simulink model "ofdm_agc_mimo"  (Simulink 7.7)
settings: Solver=VariableStepDiscrete  SolverMode=SingleTasking  StartTime=0.0  StopTime=400  RelTol=1e-3
InitFcn:
  | ofdm_agc_init
StartFcn:
  | ofdm_agc_init
values from neighbouring files (symbols this model uses):
  ltbl = ltbl(2:2049)    [ofdm_agc_init.m]
undefined symbols (not defined in the file or in its folder): gcbh, xlBlockLoadCallback, xlGetNormalizedPeriod
libraries: xbsIndex_r4 x570
(part 5 of 6)

== system ofdm_agc_mimo/Dual_channel_VIQ/AVG_I_Q3 ==
  note: Calculates the average of the I and Q channels, before taking the CPLX mag
  RESET : Inport
  CPLX_in : Inport  Port=2
  IQAvg_Len : Inport  Port=3
  ASR_I : xbsIndex_r4/Addressable Shift Register  infer_latency=on  depth=2  initVector=[0]  en=off  dbl_ovrd=off  use_behavioral_HDL=off  Optimization=Resource  use_rpm=off  block_type=addrsr
      settings: infoedit="Delay of  configurable length.  Any element  in the delay     line   can    be   addressed   and   driven    onto   the   output     port.<P><P>Hardware  notes: Implemented  using SRL16s.     If Virtex-4, Virtex-II or Spartan-3 devices are used, multiple SRLC16s are cascaded together."  xl_area=[51 0 0 102 0 0 0]  block_version=VER_STRING_GOES_HERE
  Accumulator : xbsIndex_r4/Accumulator  operation=Add  n_bits=24  overflow=Wrap  scale=1  rst=on  hasbypass=off  en=off  dbl_ovrd=off  use_behavioral_HDL=on  implementation=Fabric  block_type=accum
      settings: infoedit="Adder or subtractor-based accumulator.   Output type and binary point position match the input.<P><P>Hardware notes: When \"Reinitialize with input 'b' on reset\" is selected, the accumulator is forced to run at the system rate even if the input 'b' is running at a slower rate."  xl_area=[12 24 0 24 0 0 0]  block_version=VER_STRING_GOES_HERE
  AddSub : xbsIndex_r4/AddSub  mode=Addition  use_carryin=off  use_carryout=off  en=off  latency=0  precision=Full  arith_type=Unsigned  n_bits=8  bin_pt=2  quantization=Truncate  overflow=Wrap  dbl_ovrd=off  use_behavioral_HDL=on  hw_selection=Fabric  pipelined=off  use_rpm=on  block_type=addsub
      settings: xl_area=[10 0 0 18 0 0 0]  block_version=VER_STRING_GOES_HERE
  Convert : xbsIndex_r4/Convert  gui_display_data_type=Fixed-point  arith_type="Signed  (2's comp)"  n_bits=24  bin_pt=16  float_type=Single  exp_bits=8  fraction_bits=24  quantization=Truncate  overflow=Wrap  en=off  latency=0  dbl_ovrd=off  pipeline=off  block_type=convert
      settings: xl_area=[0 0 0 0 0 0 0]  block_version=VER_STRING_GOES_HERE
  Convert1 : xbsIndex_r4/Convert  gui_display_data_type=Fixed-point  arith_type=Unsigned  n_bits=6  bin_pt=0  float_type=Single  exp_bits=8  fraction_bits=24  quantization=Truncate  overflow=Wrap  en=off  latency=0  dbl_ovrd=off  pipeline=off  block_type=convert
      settings: xl_area=[0 0 0 0 0 0 0]  block_version=VER_STRING_GOES_HERE
  Down Sample3 : xbsIndex_r4/Down Sample  sample_ratio=4  sample_phase="Last Value of Frame  (most efficient)"  en=off  latency=1  dbl_ovrd=off  block_type=dsamp
      settings: xl_area=[3 6 0 0 0 0 0]  block_version=VER_STRING_GOES_HERE
  Mult : xbsIndex_r4/Mult  precision=User Defined  arith_type="Signed  (2's comp)"  n_bits=16  bin_pt=13  quantization=Truncate  overflow=Wrap  en=off  latency=3  dbl_ovrd=off  use_behavioral_HDL=off  opt=Speed  use_embedded=on  optimum_pipeline=off  pipeline=on  use_rpm=on  placement_style=Rectangular shape  block_type=mult
      settings: infoedit=Hardware notes: To use the internal pipeline stage of the dedicated multiplier you must select 'Pipeline for maximum performance'.  xl_area=[21 41 0 35 0 2 0]  block_version=VER_STRING_GOES_HERE
  Negate_I : xbsIndex_r4/Negate  precision=Full  arith_type=Unsigned  n_bits=8  bin_pt=2  quantization=Truncate  overflow=Wrap  en=off  latency=0  dbl_ovrd=off  block_type=negate
      settings: xl_area=[9 0 0 18 0 0 0]  block_version=VER_STRING_GOES_HERE
  Register15 : xbsIndex_r4/Register  init=0  rst=on  en=off  dbl_ovrd=off  block_type=register
      settings: xl_area=[9 17 0 0 0 0 0]  block_version=VER_STRING_GOES_HERE
  one_over_delay : xbsIndex_r4/ROM  depth=64  initVector=[1./(1:64)]  distributed_mem=Block RAM  rst=off  init_reg=0  en=off  latency=1  gui_display_data_type=Fixed-point  arith_type=Unsigned  n_bits=8  bin_pt=8  preci_type=Single  exp_width=8  frac_width=24  dbl_ovrd=off  optimize=Area  use_rpm=off  block_type=sprom
      settings: xl_area=[8 8 0 16 0 0 0]  block_version=VER_STRING_GOES_HERE
  AVG_CPLX_out : Outport
  wires:
  RESET/1 -> Accumulator/2, Register15/2
  Register15/1 -> AddSub/1, ASR_I/1
  Convert/1 -> Accumulator/1
  Negate_I/1 -> AddSub/2
  AddSub/1 -> Convert/1
  Mult/1 -> AVG_CPLX_out/1
  IQAvg_Len/1 -> Down Sample3/1
  one_over_delay/1 -> Mult/2
  Accumulator/1 -> Mult/1
  ASR_I/1 -> Negate_I/1
  CPLX_in/1 -> Register15/1
  Down Sample3/1 -> ASR_I/2, Convert1/1
  Convert1/1 -> one_over_delay/1

== system ofdm_agc_mimo/Dual_channel_VIQ/Timeshared_squarer ==
  note: Squares four parallel streams of data
  I_A : Inport
  Q_A : Inport  Port=2
  I_B : Inport  Port=3
  Q_B : Inport  Port=4
  Convert1 : xbsIndex_r4/Convert  gui_display_data_type=Fixed-point  arith_type=Unsigned  n_bits=16  bin_pt=13  float_type=Single  exp_bits=8  fraction_bits=24  quantization="Round  (unbiased: +/- Inf)"  overflow=Wrap  en=off  latency=0  dbl_ovrd=off  pipeline=off  block_type=convert
      settings: xl_area=[13 0 0 20 0 0 0]  block_version=VER_STRING_GOES_HERE
  Delay : xbsIndex_r4/Delay  rst=off  infoeditControl=Selection of Reset will increase slice count due to use of real FFs and instead of SRLs  en=off  latency=1  dbl_ovrd=off  reg_retiming=off  block_type=delay
      settings: infoedit=Hardware notes: A delay line is a chain, each link of which is an SRL16 followed by a flip-flop. If register retiming is enabled, the delay line is a chain of flip-flops.  xl_area=[8 16 0 0 0 0 0]  block_version=VER_STRING_GOES_HERE
  Down Sample{,1..3} (4 alike) : xbsIndex_r4/Down Sample  sample_ratio=4  sample_phase="Last Value of Frame  (most efficient)"  en=off  latency=1  dbl_ovrd=off  block_type=dsamp
      settings: xl_area=[8 16 0 0 0 0 0]  block_version=VER_STRING_GOES_HERE
  Mult : xbsIndex_r4/Mult  precision=Full  arith_type="Signed  (2's comp)"  n_bits=8  bin_pt=2  quantization=Truncate  overflow=Wrap  en=off  latency=2  dbl_ovrd=off  use_behavioral_HDL=off  opt=Speed  use_embedded=on  optimum_pipeline=off  pipeline=on  use_rpm=on  placement_style=Rectangular shape  block_type=mult
      settings: infoedit=Hardware notes: To use the internal pipeline stage of the dedicated multiplier you must select 'Pipeline for maximum performance'.  xl_area=[14 28 0 28 0 1 0]  block_version=VER_STRING_GOES_HERE
  Mux : xbsIndex_r4/Mux  inputs=4  en=off  latency=0  precision=Full  arith_type=Unsigned  n_bits=16  bin_pt=14  quantization=Truncate  overflow=Wrap  dbl_ovrd=off  block_type=mux
      settings: xl_area=[14 0 0 28 0 0 0]  block_version=VER_STRING_GOES_HERE
  Register{,1..3} (4 alike) : xbsIndex_r4/Register  init=0  rst=off  en=on  dbl_ovrd=off  block_type=register
      settings: xl_area=[8 16 0 0 0 0 0]  block_version=VER_STRING_GOES_HERE
  Subsystem : Subsystem
  Up Sample{,1..3} (4 alike) : xbsIndex_r4/Up Sample  sample_ratio=4  copy_samples=on  en=off  latency=0  dbl_ovrd=off  block_type=usamp
      settings: infoedit="Up samples input data.  Inserted values  can be zeros or copies of the most recent input sample.<P><P>Hardware notes: No hardware is needed if inserted values are copies of the input sample; otherwise, a mux and single bit flip-flop are used."  xl_area=[0 0 0 0 0 0 0]  block_version=VER_STRING_GOES_HERE
  I_A2 : Outport
  Q_A2 : Outport  Port=2
  I_B2 : Outport  Port=3
  Q_B2 : Outport  Port=4
  wires:
  Convert1/1 -> Register1/1, Register/1, Register2/1, Register3/1
  Delay/1 -> I_A2/1
  Down Sample3/1 -> Q_A2/1
  Down Sample2/1 -> Delay/1
  Down Sample1/1 -> Q_B2/1
  Down Sample/1 -> I_B2/1
  Up Sample2/1 -> Mux/4
  Up Sample3/1 -> Mux/5
  Up Sample1/1 -> Mux/3
  Up Sample/1 -> Mux/2
  Subsystem/4(3) -> Register3/2
  Subsystem/3(2) -> Register2/2
  Subsystem/2(1) -> Register1/2
  Subsystem/1(0) -> Register/2
  Register3/1 -> Down Sample3/1
  Register2/1 -> Down Sample2/1
  Register1/1 -> Down Sample1/1
  Register/1 -> Down Sample/1
  Subsystem/5(Counter) -> Mux/1
  Q_B/1 -> Up Sample3/1
  I_B/1 -> Up Sample2/1
  Q_A/1 -> Up Sample1/1
  I_A/1 -> Up Sample/1
  Mux/1 -> Mult/2, Mult/1
  Mult/1 -> Convert1/1

== system ofdm_agc_mimo/Registers/Read-Write Register ==
  Constant : xbsIndex_r4/Constant  const=1  gui_display_data_type=Boolean  arith_type=Boolean  n_bits=16  bin_pt=14  preci_type=Single  exp_width=8  frac_width=24  explicit_period=on  period=1  equ=P=C  opselect=C  inp2=PCIN>>17  opr=+  inp1=P  carry=CIN  dbl_ovrd=off  block_type=constant
      settings: block_version=8.2.02
  From Register : xbsIndex_r4/From Register  shared_memory_name='Bits_w'  init=0  period=1  ownership=Locally owned and initialized  gui_display_data_type=Fixed-point  arith_type=Unsigned  n_bits=10  bin_pt=0  preci_type=Single  dbl_ovrd=off  block_type=fromreg
      settings: AttributesFormatString=From Register\n<< %<shared_memory_name> >>\n%<n_bits>\n%<period>\n%<bin_pt>\n%<arith_type>\n%<ownership>\n%<init>  infoedit="Register block that reads data to a shared memory register.  Delay of one sample period."  block_version=8.2.02
  Terminator : Terminator
  To Register : xbsIndex_r4/To Register  shared_memory_name='Bits_r'  init=0  ownership=Locally owned and initialized  explicit_data_type=on  gui_display_data_type=Fixed-point  arith_type=Unsigned  n_bits=10  bin_pt=0  preci_type=Single  dbl_ovrd=off  block_type=toreg
      settings: AttributesFormatString=To Register\n<< %<shared_memory_name> >>  infoedit="Register block that writes data to a shared memory register.  Delay of one sample period."  block_version=8.2.02
  D : Outport
  wires:
  To Register/1 -> Terminator/1
  Constant/1 -> To Register/2
  From Register/1 -> To Register/1, D/1

== system ofdm_agc_mimo/dual_RSSI_preprocessor/MA ==
  RSSI_in : Inport
  M_RESET : Inport  Port=2
  RSSIAvg_Len : Inport  Port=3
  ASR : xbsIndex_r4/Addressable Shift Register  infer_latency=on  depth=2  initVector=[0]  en=off  dbl_ovrd=off  use_behavioral_HDL=off  Optimization=Resource  use_rpm=off  block_type=addrsr
      settings: infoedit="Delay of  configurable length.  Any element  in the delay     line   can    be   addressed   and   driven    onto   the   output     port.<P><P>Hardware  notes: Implemented  using SRL16s.     If Virtex-4, Virtex-II or Spartan-3 devices are used, multiple SRLC16s are cascaded together."  xl_area=[125 0 0 250 0 0 0]  block_version=VER_STRING_GOES_HERE
  Accumulator : xbsIndex_r4/Accumulator  operation=Add  n_bits=32  overflow=Flag as error  scale=1  rst=on  hasbypass=off  en=off  dbl_ovrd=off  use_behavioral_HDL=on  implementation=Fabric  block_type=accum
      settings: infoedit="Adder or subtractor-based accumulator.   Output type and binary point position match the input.<P><P>Hardware notes: When \"Reinitialize with input 'b' on reset\" is selected, the accumulator is forced to run at the system rate even if the input 'b' is running at a slower rate."  xl_area=[17 33 0 32 0 0 0]  block_version=VER_STRING_GOES_HERE
  AddSub : xbsIndex_r4/AddSub  mode=Subtraction  use_carryin=off  use_carryout=off  en=off  latency=0  precision=Full  arith_type=Unsigned  n_bits=8  bin_pt=2  quantization=Truncate  overflow=Wrap  dbl_ovrd=off  use_behavioral_HDL=on  hw_selection=Fabric  pipelined=off  use_rpm=on  block_type=addsub
      settings: xl_area=[6 0 0 11 0 0 0]  block_version=VER_STRING_GOES_HERE
  Convert : xbsIndex_r4/Convert  gui_display_data_type=Fixed-point  arith_type=Unsigned  n_bits=6  bin_pt=0  float_type=Single  exp_bits=8  fraction_bits=24  quantization=Truncate  overflow=Saturate  en=off  latency=0  dbl_ovrd=off  pipeline=off  block_type=convert
      settings: xl_area=[4 0 0 7 0 0 0]  block_version=VER_STRING_GOES_HERE
  Down Sample : xbsIndex_r4/Down Sample  sample_ratio=4  sample_phase="Last Value of Frame  (most efficient)"  en=off  latency=1  dbl_ovrd=off  block_type=dsamp
      settings: xl_area=[4 8 0 0 0 0 0]  block_version=VER_STRING_GOES_HERE
  Down Sample1 : xbsIndex_r4/Down Sample  sample_ratio=4  sample_phase="Last Value of Frame  (most efficient)"  en=off  latency=1  dbl_ovrd=off  block_type=dsamp
      settings: xl_area=[1 1 0 0 0 0 0]  block_version=VER_STRING_GOES_HERE
  Mult : xbsIndex_r4/Mult  precision=User Defined  arith_type="Signed  (2's comp)"  n_bits=18  bin_pt=0  quantization=Truncate  overflow=Wrap  en=off  latency=3  dbl_ovrd=off  use_behavioral_HDL=off  opt=Speed  use_embedded=on  optimum_pipeline=off  pipeline=on  use_rpm=on  placement_style=Rectangular shape  block_type=mult
      settings: infoedit=Hardware notes: To use the internal pipeline stage of the dedicated multiplier you must select 'Pipeline for maximum performance'.  xl_area=[26 51 0 48 0 2 0]  block_version=VER_STRING_GOES_HERE
  ROM : xbsIndex_r4/ROM  depth=64  initVector=[1./(1:64)]  distributed_mem=Block RAM  rst=off  init_reg=0  en=off  latency=1  gui_display_data_type=Fixed-point  arith_type="Signed  (2's comp)"  n_bits=16  bin_pt=14  preci_type=Single  exp_width=8  frac_width=24  dbl_ovrd=off  optimize=Area  use_rpm=off  block_type=sprom
      settings: xl_area=[20 16 0 39 0 0 0]  block_version=VER_STRING_GOES_HERE
  Register15 : xbsIndex_r4/Register  init=0  rst=on  en=off  dbl_ovrd=off  block_type=register
      settings: xl_area=[5 10 0 0 0 0 0]  block_version=VER_STRING_GOES_HERE
  Up Sample1 : xbsIndex_r4/Up Sample  sample_ratio=4  copy_samples=on  en=off  latency=0  dbl_ovrd=off  block_type=usamp
      settings: infoedit="Up samples input data.  Inserted values  can be zeros or copies of the most recent input sample.<P><P>Hardware notes: No hardware is needed if inserted values are copies of the input sample; otherwise, a mux and single bit flip-flop are used."  xl_area=[0 0 0 0 0 0 0]  block_version=VER_STRING_GOES_HERE
  Up Sample2 : xbsIndex_r4/Up Sample  sample_ratio=4  copy_samples=on  en=off  latency=0  dbl_ovrd=off  block_type=usamp
      settings: infoedit="Up samples input data.  Inserted values  can be zeros or copies of the most recent input sample.<P><P>Hardware notes: No hardware is needed if inserted values are copies of the input sample; otherwise, a mux and single bit flip-flop are used."  xl_area=[0 0 0 0 0 0 0]  block_version=VER_STRING_GOES_HERE
  4_pt_MA : Outport
  wires:
  Up Sample2/1 -> Mult/2
  Up Sample1/1 -> Mult/1
  M_RESET/1 -> Down Sample1/1
  Register15/1 -> ASR/1, AddSub/1
  Down Sample1/1 -> Register15/2, Accumulator/2
  Down Sample/1 -> ASR/2, Convert/1
  Convert/1 -> ROM/1
  ROM/1 -> Up Sample2/1
  RSSIAvg_Len/1 -> Down Sample/1
  ASR/1 -> AddSub/2
  RSSI_in/1 -> Register15/1
  Accumulator/1 -> Up Sample1/1
  Mult/1 -> 4_pt_MA/1
  AddSub/1 -> Accumulator/1

== system ofdm_agc_mimo/dual_RSSI_preprocessor/MA1 ==
  RSSI_in : Inport
  M_RESET : Inport  Port=2
  RSSIAvg_Len : Inport  Port=3
  ASR : xbsIndex_r4/Addressable Shift Register  infer_latency=on  depth=2  initVector=[0]  en=off  dbl_ovrd=off  use_behavioral_HDL=off  Optimization=Resource  use_rpm=off  block_type=addrsr
      settings: infoedit="Delay of  configurable length.  Any element  in the delay     line   can    be   addressed   and   driven    onto   the   output     port.<P><P>Hardware  notes: Implemented  using SRL16s.     If Virtex-4, Virtex-II or Spartan-3 devices are used, multiple SRLC16s are cascaded together."  xl_area=[125 0 0 250 0 0 0]  block_version=VER_STRING_GOES_HERE
  Accumulator : xbsIndex_r4/Accumulator  operation=Add  n_bits=32  overflow=Flag as error  scale=1  rst=on  hasbypass=off  en=off  dbl_ovrd=off  use_behavioral_HDL=on  implementation=Fabric  block_type=accum
      settings: infoedit="Adder or subtractor-based accumulator.   Output type and binary point position match the input.<P><P>Hardware notes: When \"Reinitialize with input 'b' on reset\" is selected, the accumulator is forced to run at the system rate even if the input 'b' is running at a slower rate."  xl_area=[17 33 0 32 0 0 0]  block_version=VER_STRING_GOES_HERE
  AddSub : xbsIndex_r4/AddSub  mode=Subtraction  use_carryin=off  use_carryout=off  en=off  latency=0  precision=Full  arith_type=Unsigned  n_bits=8  bin_pt=2  quantization=Truncate  overflow=Wrap  dbl_ovrd=off  use_behavioral_HDL=on  hw_selection=Fabric  pipelined=off  use_rpm=on  block_type=addsub
      settings: xl_area=[6 0 0 11 0 0 0]  block_version=VER_STRING_GOES_HERE
  Convert : xbsIndex_r4/Convert  gui_display_data_type=Fixed-point  arith_type=Unsigned  n_bits=6  bin_pt=0  float_type=Single  exp_bits=8  fraction_bits=24  quantization=Truncate  overflow=Saturate  en=off  latency=0  dbl_ovrd=off  pipeline=off  block_type=convert
      settings: xl_area=[4 0 0 7 0 0 0]  block_version=VER_STRING_GOES_HERE
  Down Sample : xbsIndex_r4/Down Sample  sample_ratio=4  sample_phase="Last Value of Frame  (most efficient)"  en=off  latency=1  dbl_ovrd=off  block_type=dsamp
      settings: xl_area=[4 8 0 0 0 0 0]  block_version=VER_STRING_GOES_HERE
  Down Sample1 : xbsIndex_r4/Down Sample  sample_ratio=4  sample_phase="Last Value of Frame  (most efficient)"  en=off  latency=1  dbl_ovrd=off  block_type=dsamp
      settings: xl_area=[1 1 0 0 0 0 0]  block_version=VER_STRING_GOES_HERE
  Mult : xbsIndex_r4/Mult  precision=User Defined  arith_type="Signed  (2's comp)"  n_bits=18  bin_pt=0  quantization=Truncate  overflow=Wrap  en=off  latency=3  dbl_ovrd=off  use_behavioral_HDL=off  opt=Speed  use_embedded=on  optimum_pipeline=off  pipeline=on  use_rpm=on  placement_style=Rectangular shape  block_type=mult
      settings: infoedit=Hardware notes: To use the internal pipeline stage of the dedicated multiplier you must select 'Pipeline for maximum performance'.  xl_area=[26 51 0 48 0 2 0]  block_version=VER_STRING_GOES_HERE
  ROM : xbsIndex_r4/ROM  depth=64  initVector=[1./(1:64)]  distributed_mem=Block RAM  rst=off  init_reg=0  en=off  latency=1  gui_display_data_type=Fixed-point  arith_type="Signed  (2's comp)"  n_bits=16  bin_pt=14  preci_type=Single  exp_width=8  frac_width=24  dbl_ovrd=off  optimize=Area  use_rpm=off  block_type=sprom
      settings: xl_area=[20 16 0 39 0 0 0]  block_version=VER_STRING_GOES_HERE
  Register15 : xbsIndex_r4/Register  init=0  rst=on  en=off  dbl_ovrd=off  block_type=register
      settings: xl_area=[5 10 0 0 0 0 0]  block_version=VER_STRING_GOES_HERE
  Up Sample1 : xbsIndex_r4/Up Sample  sample_ratio=4  copy_samples=on  en=off  latency=0  dbl_ovrd=off  block_type=usamp
      settings: infoedit="Up samples input data.  Inserted values  can be zeros or copies of the most recent input sample.<P><P>Hardware notes: No hardware is needed if inserted values are copies of the input sample; otherwise, a mux and single bit flip-flop are used."  xl_area=[0 0 0 0 0 0 0]  block_version=VER_STRING_GOES_HERE
  Up Sample2 : xbsIndex_r4/Up Sample  sample_ratio=4  copy_samples=on  en=off  latency=0  dbl_ovrd=off  block_type=usamp
      settings: infoedit="Up samples input data.  Inserted values  can be zeros or copies of the most recent input sample.<P><P>Hardware notes: No hardware is needed if inserted values are copies of the input sample; otherwise, a mux and single bit flip-flop are used."  xl_area=[0 0 0 0 0 0 0]  block_version=VER_STRING_GOES_HERE
  4_pt_MA : Outport
  wires:
  AddSub/1 -> Accumulator/1
  Mult/1 -> 4_pt_MA/1
  Accumulator/1 -> Up Sample1/1
  RSSI_in/1 -> Register15/1
  ASR/1 -> AddSub/2
  RSSIAvg_Len/1 -> Down Sample/1
  ROM/1 -> Up Sample2/1
  Convert/1 -> ROM/1
  Down Sample/1 -> Convert/1, ASR/2
  Down Sample1/1 -> Accumulator/2, Register15/2
  Register15/1 -> AddSub/1, ASR/1
  M_RESET/1 -> Down Sample1/1
  Up Sample1/1 -> Mult/1
  Up Sample2/1 -> Mult/2

== system ofdm_agc_mimo/AGC_A/DCO_correction/AVG_I ==
  note: Calculates the average of the I and Q channels, before taking the CPLX mag
  M_RESET : Inport
  I_in : Inport  Port=2
  Accumulator : xbsIndex_r4/Accumulator  operation=Add  n_bits=18  overflow=Wrap  scale=1  rst=on  hasbypass=off  en=off  dbl_ovrd=off  use_behavioral_HDL=on  implementation=Fabric  block_type=accum
      settings: infoedit="Adder or subtractor-based accumulator.   Output type and binary point position match the input.<P><P>Hardware notes: When \"Reinitialize with input 'b' on reset\" is selected, the accumulator is forced to run at the system rate even if the input 'b' is running at a slower rate."  xl_area=[9 18 0 18 0 0 0]  block_version=VER_STRING_GOES_HERE
  AddSub : xbsIndex_r4/AddSub  mode=Addition  use_carryin=off  use_carryout=off  en=off  latency=0  precision=Full  arith_type=Unsigned  n_bits=8  bin_pt=2  quantization=Truncate  overflow=Wrap  dbl_ovrd=off  use_behavioral_HDL=on  hw_selection=Fabric  pipelined=off  use_rpm=on  block_type=addsub
      settings: xl_area=[8 0 0 15 0 0 0]  block_version=VER_STRING_GOES_HERE
  Convert1 : xbsIndex_r4/Convert  gui_display_data_type=Fixed-point  arith_type="Signed  (2's comp)"  n_bits=15  bin_pt=14  float_type=Single  exp_bits=8  fraction_bits=24  quantization=Truncate  overflow=Wrap  en=off  latency=0  dbl_ovrd=off  pipeline=off  block_type=convert
      settings: xl_area=[0 0 0 0 0 0 0]  block_version=VER_STRING_GOES_HERE
  Delay : xbsIndex_r4/Delay  rst=off  infoeditControl=Selection of Reset will increase slice count due to use of real FFs and instead of SRLs  en=off  latency=16  dbl_ovrd=off  reg_retiming=off  block_type=delay
      settings: infoedit=Hardware notes: A delay line is a chain, each link of which is an SRL16 followed by a flip-flop. If register retiming is enabled, the delay line is a chain of flip-flops.  xl_area=[7 14 0 14 0 0 0]  block_version=VER_STRING_GOES_HERE
  Negate_I : xbsIndex_r4/Negate  precision=Full  arith_type=Unsigned  n_bits=8  bin_pt=2  quantization=Truncate  overflow=Wrap  en=off  latency=0  dbl_ovrd=off  block_type=negate
      settings: xl_area=[8 0 0 15 0 0 0]  block_version=VER_STRING_GOES_HERE
  Register15 : xbsIndex_r4/Register  init=0  rst=on  en=off  dbl_ovrd=off  block_type=register
      settings: xl_area=[7 14 0 0 0 0 0]  block_version=VER_STRING_GOES_HERE
  Scale : xbsIndex_r4/Scale  scale_factor=-4  dbl_ovrd=off  block_type=scale
      settings: infoedit=Scales input by a power of two by adjusting the binary point position.<P><P>Hardware notes: In hardware this block costs nothing.  block_version=VER_STRING_GOES_HERE
  AVG_I_out : Outport
  wires:
  Convert1/1 -> AVG_I_out/1
  Scale/1 -> Convert1/1
  M_RESET/1 -> Accumulator/2, Register15/2
  Register15/1 -> Delay/1, AddSub/1
  Negate_I/1 -> AddSub/2
  AddSub/1 -> Accumulator/1
  Accumulator/1 -> Scale/1
  Delay/1 -> Negate_I/1
  I_in/1 -> Register15/1

== system ofdm_agc_mimo/AGC_A/DCO_correction/AVG_Q ==
  note: Calculates the average of the I and Q channels, before taking the CPLX mag
  M_RESET : Inport
  I_in : Inport  Port=2
  Accumulator : xbsIndex_r4/Accumulator  operation=Add  n_bits=18  overflow=Wrap  scale=1  rst=on  hasbypass=off  en=off  dbl_ovrd=off  use_behavioral_HDL=on  implementation=Fabric  block_type=accum
      settings: infoedit="Adder or subtractor-based accumulator.   Output type and binary point position match the input.<P><P>Hardware notes: When \"Reinitialize with input 'b' on reset\" is selected, the accumulator is forced to run at the system rate even if the input 'b' is running at a slower rate."  xl_area=[9 18 0 18 0 0 0]  block_version=VER_STRING_GOES_HERE
  AddSub : xbsIndex_r4/AddSub  mode=Addition  use_carryin=off  use_carryout=off  en=off  latency=0  precision=Full  arith_type=Unsigned  n_bits=8  bin_pt=2  quantization=Truncate  overflow=Wrap  dbl_ovrd=off  use_behavioral_HDL=on  hw_selection=Fabric  pipelined=off  use_rpm=on  block_type=addsub
      settings: xl_area=[8 0 0 15 0 0 0]  block_version=VER_STRING_GOES_HERE
  Convert1 : xbsIndex_r4/Convert  gui_display_data_type=Fixed-point  arith_type="Signed  (2's comp)"  n_bits=15  bin_pt=14  float_type=Single  exp_bits=8  fraction_bits=24  quantization=Truncate  overflow=Wrap  en=off  latency=0  dbl_ovrd=off  pipeline=off  block_type=convert
      settings: xl_area=[0 0 0 0 0 0 0]  block_version=VER_STRING_GOES_HERE
  Delay : xbsIndex_r4/Delay  rst=off  infoeditControl=Selection of Reset will increase slice count due to use of real FFs and instead of SRLs  en=off  latency=16  dbl_ovrd=off  reg_retiming=off  block_type=delay
      settings: infoedit=Hardware notes: A delay line is a chain, each link of which is an SRL16 followed by a flip-flop. If register retiming is enabled, the delay line is a chain of flip-flops.  xl_area=[7 14 0 14 0 0 0]  block_version=VER_STRING_GOES_HERE
  Negate_I : xbsIndex_r4/Negate  precision=Full  arith_type=Unsigned  n_bits=8  bin_pt=2  quantization=Truncate  overflow=Wrap  en=off  latency=0  dbl_ovrd=off  block_type=negate
      settings: xl_area=[8 0 0 15 0 0 0]  block_version=VER_STRING_GOES_HERE
  Register15 : xbsIndex_r4/Register  init=0  rst=on  en=off  dbl_ovrd=off  block_type=register
      settings: xl_area=[7 14 0 0 0 0 0]  block_version=VER_STRING_GOES_HERE
  Scale : xbsIndex_r4/Scale  scale_factor=-4  dbl_ovrd=off  block_type=scale
      settings: infoedit=Scales input by a power of two by adjusting the binary point position.<P><P>Hardware notes: In hardware this block costs nothing.  block_version=VER_STRING_GOES_HERE
  AVG_I_out : Outport
  wires:
  I_in/1 -> Register15/1
  Delay/1 -> Negate_I/1
  Accumulator/1 -> Scale/1
  AddSub/1 -> Accumulator/1
  Negate_I/1 -> AddSub/2
  Register15/1 -> Delay/1, AddSub/1
  M_RESET/1 -> Register15/2, Accumulator/2
  Scale/1 -> Convert1/1
  Convert1/1 -> AVG_I_out/1

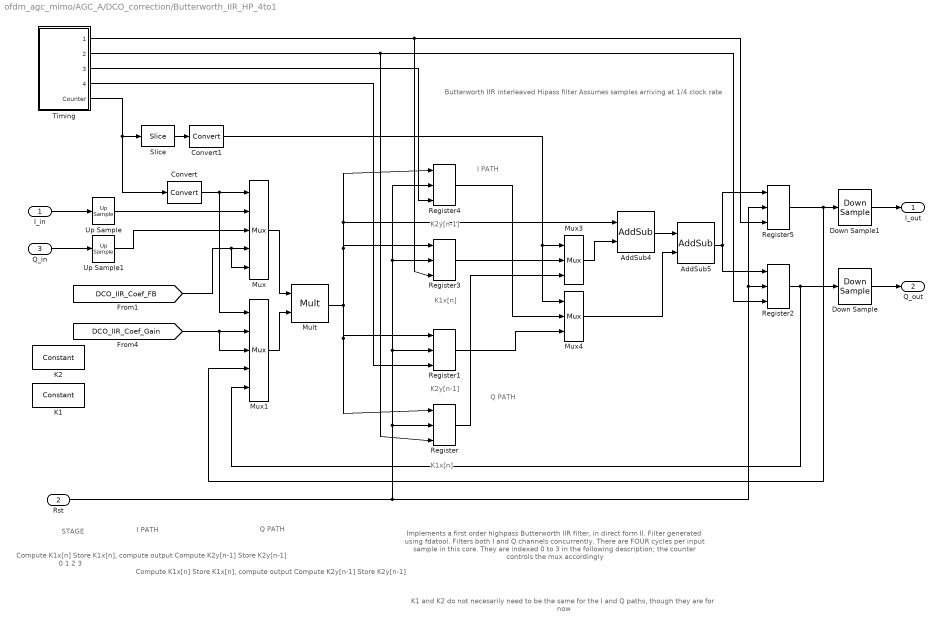
== system ofdm_agc_mimo/AGC_A/DCO_correction/Butterworth_IIR_HP_4to1 ==
  note: K1x[n]
  note: K2y[n-1]
  note: K1x[n]
  note: K2y[n-1]
  note: Implements a first order highpass Butterworth IIR filter,
      | in direct form II.  Filter generated using fdatool.
      | Filters both I and Q channels concurrently.
      |
      | There are FOUR cycles per input sample in this core.  They
      | are indexed 0 to 3 in the following description; the counter
      | controls the mux accordingly
  note: I PATH
  note: Q PATH
  note: 0
      | 1
      | 2
      | 3
  note: Compute K1x[n]
      | Store K1x[n], compute output
      | Compute K2y[n-1]
      | Store K2y[n-1]
  note: Compute K1x[n]
      | Store K1x[n], compute output
      | Compute K2y[n-1]
      | Store K2y[n-1]
  note: STAGE
  note: Q PATH
  note: I PATH
  note: K1 and K2 do not necesarily need to be the same
      | for the I and Q paths, though they are for now
  note: Butterworth IIR interleaved Hipass filter
      | Assumes samples arriving at 1/4 clock rate
  I_in : Inport
  Rst : Inport  Port=2
  Q_in : Inport  Port=3
  AddSub4 : xbsIndex_r4/AddSub  mode=Subtraction  use_carryin=off  use_carryout=off  en=off  latency=0  precision=Full  arith_type=Unsigned  n_bits=8  bin_pt=2  quantization=Truncate  overflow=Wrap  dbl_ovrd=off  use_behavioral_HDL=on  hw_selection=Fabric  pipelined=off  use_rpm=on  block_type=addsub
      settings: xl_area=[9 0 0 17 0 0 0]  block_version=VER_STRING_GOES_HERE
  AddSub5 : xbsIndex_r4/AddSub  mode=Subtraction  use_carryin=off  use_carryout=off  en=off  latency=0  precision=Full  arith_type=Unsigned  n_bits=8  bin_pt=2  quantization=Truncate  overflow=Wrap  dbl_ovrd=off  use_behavioral_HDL=on  hw_selection=Fabric  pipelined=off  use_rpm=on  block_type=addsub
      settings: xl_area=[9 0 0 18 0 0 0]  block_version=VER_STRING_GOES_HERE
  Convert : xbsIndex_r4/Convert  gui_display_data_type=Fixed-point  arith_type=Unsigned  n_bits=2  bin_pt=0  float_type=Single  exp_bits=8  fraction_bits=24  quantization=Truncate  overflow=Wrap  en=off  latency=0  dbl_ovrd=off  pipeline=off  block_type=convert
      settings: xl_area=[0 0 0 0 0 0 0]  block_version=VER_STRING_GOES_HERE
  Convert1 : xbsIndex_r4/Convert  gui_display_data_type=Fixed-point  arith_type=Unsigned  n_bits=1  bin_pt=0  float_type=Single  exp_bits=8  fraction_bits=24  quantization=Truncate  overflow=Wrap  en=off  latency=0  dbl_ovrd=off  pipeline=off  block_type=convert
      settings: xl_area=[0 0 0 0 0 0 0]  block_version=VER_STRING_GOES_HERE
  Down Sample : xbsIndex_r4/Down Sample  sample_ratio=4  sample_phase="Last Value of Frame  (most efficient)"  en=off  latency=1  dbl_ovrd=off  block_type=dsamp
      settings: xl_area=[9 18 0 0 0 0 0]  block_version=VER_STRING_GOES_HERE
  Down Sample1 : xbsIndex_r4/Down Sample  sample_ratio=4  sample_phase="Last Value of Frame  (most efficient)"  en=off  latency=1  dbl_ovrd=off  block_type=dsamp
      settings: xl_area=[9 18 0 0 0 0 0]  block_version=VER_STRING_GOES_HERE
  K1 : xbsIndex_r4/Constant  const=0.99375596495365714  gui_display_data_type=Fixed-point  arith_type=Unsigned  n_bits=18  bin_pt=17  preci_type=Single  exp_width=8  frac_width=24  explicit_period=off  period=1  equ=P=C  opselect=C  inp2=PCIN>>17  opr=+  inp1=P  carry=CIN  dbl_ovrd=off  block_type=constant
      settings: block_version=VER_STRING_GOES_HERE
  K2 : xbsIndex_r4/Constant  const=-0.98751192990731429  gui_display_data_type=Fixed-point  arith_type=Signed (2's comp)  n_bits=18  bin_pt=17  preci_type=Single  exp_width=8  frac_width=24  explicit_period=off  period=1  equ=P=C  opselect=C  inp2=PCIN>>17  opr=+  inp1=P  carry=CIN  dbl_ovrd=off  block_type=constant
      settings: block_version=VER_STRING_GOES_HERE
  Mult : xbsIndex_r4/Mult  precision=User Defined  arith_type="Signed  (2's comp)"  n_bits=36  bin_pt=32  quantization=Truncate  overflow=Wrap  en=off  latency=1  dbl_ovrd=off  use_behavioral_HDL=off  opt=Speed  use_embedded=on  optimum_pipeline=off  pipeline=off  use_rpm=on  placement_style=Rectangular shape  block_type=mult
      settings: infoedit=Hardware notes: To use the internal pipeline stage of the dedicated multiplier you must select 'Pipeline for maximum performance'.  xl_area=[56 18 0 109 0 4 0]  block_version=VER_STRING_GOES_HERE
  Mux : xbsIndex_r4/Mux  inputs=4  en=off  latency=0  precision=Full  arith_type="Signed  (2's comp)"  n_bits=8  bin_pt=2  quantization=Truncate  overflow=Wrap  dbl_ovrd=off  block_type=mux
      settings: xl_area=[20 0 0 40 0 0 0]  block_version=VER_STRING_GOES_HERE
  Mux1 : xbsIndex_r4/Mux  inputs=4  en=off  latency=0  precision=User Defined  arith_type="Signed  (2's comp)"  n_bits=36  bin_pt=32  quantization=Truncate  overflow=Wrap  dbl_ovrd=off  block_type=mux
      settings: xl_area=[18 0 0 36 0 0 0]  block_version=VER_STRING_GOES_HERE
  Mux3 : xbsIndex_r4/Mux  inputs=2  en=off  latency=0  precision=Full  arith_type="Signed  (2's comp)"  n_bits=8  bin_pt=2  quantization=Truncate  overflow=Wrap  dbl_ovrd=off  block_type=mux
      settings: xl_area=[8 0 0 16 0 0 0]  block_version=VER_STRING_GOES_HERE
  Mux4 : xbsIndex_r4/Mux  inputs=2  en=off  latency=0  precision=Full  arith_type="Signed  (2's comp)"  n_bits=8  bin_pt=2  quantization=Truncate  overflow=Wrap  dbl_ovrd=off  block_type=mux
      settings: xl_area=[8 0 0 16 0 0 0]  block_version=VER_STRING_GOES_HERE
  Register{,1..5} (6 alike) : xbsIndex_r4/Register  init=0  rst=on  en=on  dbl_ovrd=off  block_type=register
      Register settings: xl_area=[8 16 0 0 0 0 0]  block_version=VER_STRING_GOES_HERE
      Register1 settings: xl_area=[8 16 0 0 0 0 0]  block_version=VER_STRING_GOES_HERE
      Register2 settings: xl_area=[9 18 0 0 0 0 0]  block_version=VER_STRING_GOES_HERE
      Register3 settings: xl_area=[8 16 0 0 0 0 0]  block_version=VER_STRING_GOES_HERE
      Register4 settings: xl_area=[8 16 0 0 0 0 0]  block_version=VER_STRING_GOES_HERE
      Register5 settings: xl_area=[9 18 0 0 0 0 0]  block_version=VER_STRING_GOES_HERE
  Slice : xbsIndex_r4/Slice  nbits=1  boolean_output=off  mode=Lower Bit Location + Width  bit1=1  base1=MSB of Input  bit0=1  base0=LSB of Input  dbl_ovrd=off  block_type=slice
      settings: infoedit="Extracts a given range of bits from each input sample and presents it at the output.  The output type is ordinarily unsigned with binary point at zero, but can be Boolean when the slice is one bit wide.<P><P>Hardware notes: In hardware this block costs nothing."  block_version=VER_STRING_GOES_HERE
  Timing : Subsystem
  Up Sample : xbsIndex_r4/Up Sample  sample_ratio=4  copy_samples=on  en=off  latency=0  dbl_ovrd=off  block_type=usamp
      settings: infoedit="Up samples input data.  Inserted values  can be zeros or copies of the most recent input sample.<P><P>Hardware notes: No hardware is needed if inserted values are copies of the input sample; otherwise, a mux and single bit flip-flop are used."  xl_area=[0 0 0 0 0 0 0]  block_version=VER_STRING_GOES_HERE
  Up Sample1 : xbsIndex_r4/Up Sample  sample_ratio=4  copy_samples=on  en=off  latency=0  dbl_ovrd=off  block_type=usamp
      settings: infoedit="Up samples input data.  Inserted values  can be zeros or copies of the most recent input sample.<P><P>Hardware notes: No hardware is needed if inserted values are copies of the input sample; otherwise, a mux and single bit flip-flop are used."  xl_area=[0 0 0 0 0 0 0]  block_version=VER_STRING_GOES_HERE
  I_out : Outport
  Q_out : Outport  Port=2
  wires:
  I_in/1 -> Up Sample/1
  Up Sample/1 -> Mux/2
  Mux/1 -> Mult/1
  Mux1/1 -> Mult/2
  Mult/1 -> Register/1, Register1/1, Register3/1, Register4/1, AddSub4/1
  Register/1 -> Mux3/3
  Convert/1 -> Mux/1, Mux1/1
  Register2/1 -> Down Sample/1, Mux1/5
  Down Sample/1 -> Q_out/1
  Q_in/1 -> Up Sample1/1
  [DCO_IIR_Coef_Gain] -> Mux1/2, Mux1/3
  Up Sample1/1 -> Mux/3
  [DCO_IIR_Coef_FB] -> Mux/4, Mux/5
  Timing/5(Counter) -> Convert/1, Slice/1
  Register3/1 -> Mux3/2
  Register5/1 -> Down Sample1/1, Mux1/4
  Down Sample1/1 -> I_out/1
  Slice/1 -> Convert1/1
  AddSub4/1 -> AddSub5/1
  Mux4/1 -> AddSub5/2
  Mux3/1 -> AddSub4/2
  AddSub5/1 -> Register5/1, Register2/1
  Register4/1 -> Mux4/2
  Register1/1 -> Mux4/3
  Convert1/1 -> Mux4/1, Mux3/1
  Timing/1(1) -> Register3/3, Register5/3
  Timing/3(3) -> Register4/3
  Timing/2(2) -> Register/3, Register2/3
  Timing/4(4) -> Register1/3
  Rst/1 -> Register4/2, Register3/2, Register1/2, Register/2, Register5/2, Register2/2

== system ofdm_agc_mimo/AGC_A/DCO_correction/SR Latch ==
  R : Inport
  S : Inport  Port=2
  Constant : xbsIndex_r4/Constant  const=1  gui_display_data_type=Fixed-point  arith_type=Boolean  n_bits=1  bin_pt=0  preci_type=Single  exp_width=8  frac_width=24  explicit_period=off  period=1  equ=P=C  opselect=C  inp2=PCIN>>17  opr=+  inp1=P  carry=CIN  dbl_ovrd=off  block_type=constant
      settings: block_version=VER_STRING_GOES_HERE
  Register2 : xbsIndex_r4/Register  init=0  rst=on  en=on  dbl_ovrd=off  block_type=register
      settings: xl_area=[1 1 0 0 0 0 0]  block_version=VER_STRING_GOES_HERE
  Out1 : Outport
  wires:
  Register2/1 -> Out1/1
  Constant/1 -> Register2/1
  R/1 -> Register2/2
  S/1 -> Register2/3

== system ofdm_agc_mimo/AGC_A/DCO_correction/Subsystem ==
  US_IN : Inport
  Constant : xbsIndex_r4/Constant  const=1  gui_display_data_type=Fixed-point  arith_type=Boolean  n_bits=16  bin_pt=14  preci_type=Single  exp_width=8  frac_width=24  explicit_period=off  period=1  equ=P=C  opselect=C  inp2=PCIN>>17  opr=+  inp1=P  carry=CIN  dbl_ovrd=off  block_type=constant
      settings: block_version=VER_STRING_GOES_HERE
  Delay : xbsIndex_r4/Delay  rst=off  infoeditControl=Selection of Reset will increase slice count due to use of real FFs and instead of SRLs  en=off  latency=1  dbl_ovrd=off  reg_retiming=off  block_type=delay
      settings: infoedit=Hardware notes: A delay line is a chain, each link of which is an SRL16 followed by a flip-flop. If register retiming is enabled, the delay line is a chain of flip-flops.  xl_area=[1 1 0 0 0 0 0]  block_version=VER_STRING_GOES_HERE
  Down Sample : xbsIndex_r4/Down Sample  sample_ratio=4  sample_phase="Last Value of Frame  (most efficient)"  en=off  latency=1  dbl_ovrd=off  block_type=dsamp
      settings: xl_area=[1 1 0 0 0 0 0]  block_version=VER_STRING_GOES_HERE
  Inverter : xbsIndex_r4/Inverter  en=off  latency=0  dbl_ovrd=off  block_type=inv
      settings: xl_area=[0 0 0 0 0 0 0]  block_version=VER_STRING_GOES_HERE
  Logical : xbsIndex_r4/Logical  logical_function=AND  inputs=2  en=off  latency=0  precision=Full  arith_type=Unsigned  n_bits=16  bin_pt=0  align_bp=on  dbl_ovrd=off  block_type=logical
      settings: xl_area=[1 0 0 1 0 0 0]  block_version=VER_STRING_GOES_HERE
  Register : xbsIndex_r4/Register  init=0  rst=on  en=on  dbl_ovrd=off  block_type=register
      settings: xl_area=[1 1 0 0 0 0 0]  block_version=VER_STRING_GOES_HERE
  Up Sample : xbsIndex_r4/Up Sample  sample_ratio=4  copy_samples=on  en=off  latency=0  dbl_ovrd=off  block_type=usamp
      settings: infoedit="Up samples input data.  Inserted values  can be zeros or copies of the most recent input sample.<P><P>Hardware notes: No hardware is needed if inserted values are copies of the input sample; otherwise, a mux and single bit flip-flop are used."  xl_area=[0 0 0 0 0 0 0]  block_version=VER_STRING_GOES_HERE
  DS_OUT : Outport
  wires:
  US_IN/1 -> Register/3
  Constant/1 -> Register/1
  Register/1 -> Down Sample/1
  Down Sample/1 -> Delay/1, Logical/1, DS_OUT/1
  Inverter/1 -> Logical/2
  Delay/1 -> Inverter/1
  Logical/1 -> Up Sample/1
  Up Sample/1 -> Register/2

== system ofdm_agc_mimo/AGC_A/DCO_correction/Timing ==
  note: 3, 48, 64, 70
      | 0x46403003
  EN : Inport
  RST : Inport  Port=2
  Timing : Inport  Port=3
  Counter : xbsIndex_r4/Counter  cnt_type=Free Running  cnt_to=Inf  operation=Up  start_count=0  cnt_by_val=1  arith_type=Unsigned  n_bits=8  bin_pt=0  load_pin=off  rst=on  en=on  explicit_period=on  period=4  dbl_ovrd=off  use_behavioral_HDL=off  implementation=Fabric  use_rpm=on  block_type=counter
      settings: xl_area=[5 8 0 8 0 0 0]  block_version=VER_STRING_GOES_HERE
  Demux : Subsystem
  Down Sample : xbsIndex_r4/Down Sample  sample_ratio=4  sample_phase=First Value of Frame  en=off  latency=0  dbl_ovrd=off  block_type=dsamp
      settings: xl_area=[33 33 0 32 0 0 0]  block_version=VER_STRING_GOES_HERE
  Inverter : xbsIndex_r4/Inverter  en=off  latency=0  dbl_ovrd=off  block_type=inv
      settings: xl_area=[0 0 0 0 0 0 0]  block_version=VER_STRING_GOES_HERE
  Logical : xbsIndex_r4/Logical  logical_function=AND  inputs=2  en=off  latency=0  precision=Full  arith_type=Unsigned  n_bits=8  bin_pt=2  align_bp=on  dbl_ovrd=off  block_type=logical
      settings: xl_area=[1 0 0 1 0 0 0]  block_version=VER_STRING_GOES_HERE
  Logical1 : xbsIndex_r4/Logical  logical_function=OR  inputs=2  en=off  latency=0  precision=Full  arith_type=Unsigned  n_bits=8  bin_pt=2  align_bp=on  dbl_ovrd=off  block_type=logical
      settings: xl_area=[1 0 0 1 0 0 0]  block_version=VER_STRING_GOES_HERE
  Relational{,1..3} (4 alike) : xbsIndex_r4/Relational  mode=a=b  en=off  latency=0  dbl_ovrd=off  block_type=relational
      settings: xl_area=[2 0 0 4 0 0 0]  block_version=VER_STRING_GOES_HERE
  3 : Outport
  both_48_64 : Outport  Port=2
  70 : Outport  Port=3
  wires:
  Counter/1 -> Relational/1, Relational1/1, Relational3/1, Relational2/1
  Logical/1 -> Counter/2
  RST/1 -> Counter/1
  Demux/4(Hi) -> Relational3/2
  Demux/3(MH) -> Relational2/2
  Demux/2(ML) -> Relational1/2
  Demux/1(Lo) -> Relational/2
  Relational/1 -> 3/1
  Relational3/1 -> 70/1, Inverter/1
  EN/1 -> Logical/1
  Inverter/1 -> Logical/2
  Logical1/1 -> both_48_64/1
  Relational1/1 -> Logical1/1
  Relational2/1 -> Logical1/2
  Timing/1 -> Down Sample/1
  Down Sample/1 -> Demux/1(In1)

== system ofdm_agc_mimo/AGC_A/RF_setting/8bit_slicer1 ==
  In1 : Inport
  Convert4 : xbsIndex_r4/Convert  gui_display_data_type=Fixed-point  arith_type="Signed  (2's comp)"  n_bits=8  bin_pt=0  float_type=Single  exp_bits=8  fraction_bits=24  quantization=Truncate  overflow=Wrap  en=off  latency=0  dbl_ovrd=off  pipeline=off  block_type=convert
      settings: xl_area=[0 0 0 0 0 0 0]  block_version=VER_STRING_GOES_HERE
  Convert5 : xbsIndex_r4/Convert  gui_display_data_type=Fixed-point  arith_type="Signed  (2's comp)"  n_bits=8  bin_pt=0  float_type=Single  exp_bits=8  fraction_bits=24  quantization=Truncate  overflow=Wrap  en=off  latency=0  dbl_ovrd=off  pipeline=off  block_type=convert
      settings: xl_area=[0 0 0 0 0 0 0]  block_version=VER_STRING_GOES_HERE
  Convert6 : xbsIndex_r4/Convert  gui_display_data_type=Fixed-point  arith_type="Signed  (2's comp)"  n_bits=8  bin_pt=0  float_type=Single  exp_bits=8  fraction_bits=24  quantization=Truncate  overflow=Wrap  en=off  latency=0  dbl_ovrd=off  pipeline=off  block_type=convert
      settings: xl_area=[0 0 0 0 0 0 0]  block_version=VER_STRING_GOES_HERE
  Slice1 : xbsIndex_r4/Slice  nbits=8  boolean_output=off  mode=Lower Bit Location + Width  bit1=0  base1=MSB of Input  bit0=0  base0=LSB of Input  dbl_ovrd=off  block_type=slice
      settings: infoedit="Extracts a given range of bits from each input sample and presents it at the output.  The output type is ordinarily unsigned with binary point at zero, but can be Boolean when the slice is one bit wide.<P><P>Hardware notes: In hardware this block costs nothing."  block_version=VER_STRING_GOES_HERE
  Slice2 : xbsIndex_r4/Slice  nbits=8  boolean_output=off  mode=Lower Bit Location + Width  bit1=0  base1=MSB of Input  bit0=8  base0=LSB of Input  dbl_ovrd=off  block_type=slice
      settings: infoedit="Extracts a given range of bits from each input sample and presents it at the output.  The output type is ordinarily unsigned with binary point at zero, but can be Boolean when the slice is one bit wide.<P><P>Hardware notes: In hardware this block costs nothing."  block_version=VER_STRING_GOES_HERE
  Slice3 : xbsIndex_r4/Slice  nbits=8  boolean_output=off  mode=Lower Bit Location + Width  bit1=0  base1=MSB of Input  bit0=16  base0=LSB of Input  dbl_ovrd=off  block_type=slice
      settings: infoedit="Extracts a given range of bits from each input sample and presents it at the output.  The output type is ordinarily unsigned with binary point at zero, but can be Boolean when the slice is one bit wide.<P><P>Hardware notes: In hardware this block costs nothing."  block_version=VER_STRING_GOES_HERE
  Out1 : Outport
  Out2 : Outport  Port=2
  Out3 : Outport  Port=3
  wires:
  In1/1 -> Slice1/1, Slice2/1, Slice3/1
  Slice1/1 -> Convert4/1
  Slice2/1 -> Convert5/1
  Slice3/1 -> Convert6/1
  Convert4/1 -> Out1/1
  Convert5/1 -> Out2/1
  Convert6/1 -> Out3/1

== system ofdm_agc_mimo/AGC_A/Stage_UD/RisingEdge ==
  IN : Inport
  Delay : xbsIndex_r4/Delay  rst=off  infoeditControl=Selection of Reset will increase slice count due to use of real FFs and instead of SRLs  en=off  latency=1  dbl_ovrd=off  reg_retiming=off  block_type=delay
      settings: infoedit=Hardware notes: A delay line is a chain, each link of which is an SRL16 followed by a flip-flop. If register retiming is enabled, the delay line is a chain of flip-flops.  xl_area=[1 1 0 0 0 0 0]  block_version=VER_STRING_GOES_HERE
  Inverter : xbsIndex_r4/Inverter  en=off  latency=0  dbl_ovrd=off  block_type=inv
      settings: xl_area=[0 0 0 0 0 0 0]  block_version=VER_STRING_GOES_HERE
  Logical : xbsIndex_r4/Logical  logical_function=AND  inputs=2  en=off  latency=0  precision=Full  arith_type=Unsigned  n_bits=16  bin_pt=0  align_bp=on  dbl_ovrd=off  block_type=logical
      settings: xl_area=[1 0 0 1 0 0 0]  block_version=VER_STRING_GOES_HERE
  Edge : Outport
  wires:
  Logical/1 -> Edge/1
  Delay/1 -> Logical/2
  Inverter/1 -> Delay/1
  IN/1 -> Logical/1, Inverter/1

== system ofdm_agc_mimo/AGC_B/DCO_correction/AVG_I ==
  note: Calculates the average of the I and Q channels, before taking the CPLX mag
  M_RESET : Inport
  I_in : Inport  Port=2
  Accumulator : xbsIndex_r4/Accumulator  operation=Add  n_bits=18  overflow=Wrap  scale=1  rst=on  hasbypass=off  en=off  dbl_ovrd=off  use_behavioral_HDL=on  implementation=Fabric  block_type=accum
      settings: infoedit="Adder or subtractor-based accumulator.   Output type and binary point position match the input.<P><P>Hardware notes: When \"Reinitialize with input 'b' on reset\" is selected, the accumulator is forced to run at the system rate even if the input 'b' is running at a slower rate."  xl_area=[9 18 0 18 0 0 0]  block_version=VER_STRING_GOES_HERE
  AddSub : xbsIndex_r4/AddSub  mode=Addition  use_carryin=off  use_carryout=off  en=off  latency=0  precision=Full  arith_type=Unsigned  n_bits=8  bin_pt=2  quantization=Truncate  overflow=Wrap  dbl_ovrd=off  use_behavioral_HDL=on  hw_selection=Fabric  pipelined=off  use_rpm=on  block_type=addsub
      settings: xl_area=[8 0 0 15 0 0 0]  block_version=VER_STRING_GOES_HERE
  Convert1 : xbsIndex_r4/Convert  gui_display_data_type=Fixed-point  arith_type="Signed  (2's comp)"  n_bits=15  bin_pt=14  float_type=Single  exp_bits=8  fraction_bits=24  quantization=Truncate  overflow=Wrap  en=off  latency=0  dbl_ovrd=off  pipeline=off  block_type=convert
      settings: xl_area=[0 0 0 0 0 0 0]  block_version=VER_STRING_GOES_HERE
  Delay : xbsIndex_r4/Delay  rst=off  infoeditControl=Selection of Reset will increase slice count due to use of real FFs and instead of SRLs  en=off  latency=16  dbl_ovrd=off  reg_retiming=off  block_type=delay
      settings: infoedit=Hardware notes: A delay line is a chain, each link of which is an SRL16 followed by a flip-flop. If register retiming is enabled, the delay line is a chain of flip-flops.  xl_area=[7 14 0 14 0 0 0]  block_version=VER_STRING_GOES_HERE
  Negate_I : xbsIndex_r4/Negate  precision=Full  arith_type=Unsigned  n_bits=8  bin_pt=2  quantization=Truncate  overflow=Wrap  en=off  latency=0  dbl_ovrd=off  block_type=negate
      settings: xl_area=[8 0 0 15 0 0 0]  block_version=VER_STRING_GOES_HERE
  Register15 : xbsIndex_r4/Register  init=0  rst=on  en=off  dbl_ovrd=off  block_type=register
      settings: xl_area=[7 14 0 0 0 0 0]  block_version=VER_STRING_GOES_HERE
  Scale : xbsIndex_r4/Scale  scale_factor=-4  dbl_ovrd=off  block_type=scale
      settings: infoedit=Scales input by a power of two by adjusting the binary point position.<P><P>Hardware notes: In hardware this block costs nothing.  block_version=VER_STRING_GOES_HERE
  AVG_I_out : Outport
  wires:
  Convert1/1 -> AVG_I_out/1
  Scale/1 -> Convert1/1
  M_RESET/1 -> Accumulator/2, Register15/2
  Register15/1 -> Delay/1, AddSub/1
  Negate_I/1 -> AddSub/2
  AddSub/1 -> Accumulator/1
  Accumulator/1 -> Scale/1
  Delay/1 -> Negate_I/1
  I_in/1 -> Register15/1

== system ofdm_agc_mimo/AGC_B/DCO_correction/AVG_Q ==
  note: Calculates the average of the I and Q channels, before taking the CPLX mag
  M_RESET : Inport
  I_in : Inport  Port=2
  Accumulator : xbsIndex_r4/Accumulator  operation=Add  n_bits=18  overflow=Wrap  scale=1  rst=on  hasbypass=off  en=off  dbl_ovrd=off  use_behavioral_HDL=on  implementation=Fabric  block_type=accum
      settings: infoedit="Adder or subtractor-based accumulator.   Output type and binary point position match the input.<P><P>Hardware notes: When \"Reinitialize with input 'b' on reset\" is selected, the accumulator is forced to run at the system rate even if the input 'b' is running at a slower rate."  xl_area=[9 18 0 18 0 0 0]  block_version=VER_STRING_GOES_HERE
  AddSub : xbsIndex_r4/AddSub  mode=Addition  use_carryin=off  use_carryout=off  en=off  latency=0  precision=Full  arith_type=Unsigned  n_bits=8  bin_pt=2  quantization=Truncate  overflow=Wrap  dbl_ovrd=off  use_behavioral_HDL=on  hw_selection=Fabric  pipelined=off  use_rpm=on  block_type=addsub
      settings: xl_area=[8 0 0 15 0 0 0]  block_version=VER_STRING_GOES_HERE
  Convert1 : xbsIndex_r4/Convert  gui_display_data_type=Fixed-point  arith_type="Signed  (2's comp)"  n_bits=15  bin_pt=14  float_type=Single  exp_bits=8  fraction_bits=24  quantization=Truncate  overflow=Wrap  en=off  latency=0  dbl_ovrd=off  pipeline=off  block_type=convert
      settings: xl_area=[0 0 0 0 0 0 0]  block_version=VER_STRING_GOES_HERE
  Delay : xbsIndex_r4/Delay  rst=off  infoeditControl=Selection of Reset will increase slice count due to use of real FFs and instead of SRLs  en=off  latency=16  dbl_ovrd=off  reg_retiming=off  block_type=delay
      settings: infoedit=Hardware notes: A delay line is a chain, each link of which is an SRL16 followed by a flip-flop. If register retiming is enabled, the delay line is a chain of flip-flops.  xl_area=[7 14 0 14 0 0 0]  block_version=VER_STRING_GOES_HERE
  Negate_I : xbsIndex_r4/Negate  precision=Full  arith_type=Unsigned  n_bits=8  bin_pt=2  quantization=Truncate  overflow=Wrap  en=off  latency=0  dbl_ovrd=off  block_type=negate
      settings: xl_area=[8 0 0 15 0 0 0]  block_version=VER_STRING_GOES_HERE
  Register15 : xbsIndex_r4/Register  init=0  rst=on  en=off  dbl_ovrd=off  block_type=register
      settings: xl_area=[7 14 0 0 0 0 0]  block_version=VER_STRING_GOES_HERE
  Scale : xbsIndex_r4/Scale  scale_factor=-4  dbl_ovrd=off  block_type=scale
      settings: infoedit=Scales input by a power of two by adjusting the binary point position.<P><P>Hardware notes: In hardware this block costs nothing.  block_version=VER_STRING_GOES_HERE
  AVG_I_out : Outport
  wires:
  I_in/1 -> Register15/1
  Delay/1 -> Negate_I/1
  Accumulator/1 -> Scale/1
  AddSub/1 -> Accumulator/1
  Negate_I/1 -> AddSub/2
  Register15/1 -> Delay/1, AddSub/1
  M_RESET/1 -> Register15/2, Accumulator/2
  Scale/1 -> Convert1/1
  Convert1/1 -> AVG_I_out/1
